simulink model "lab_1_v3"  (R2014a)
settings: Solver=ode3  StartTime=0.0  StopTime=inf  RelTol=1e-3
values from neighbouring files (symbols this model uses):
  a = 1    [aaa.m]    (also in forward.m = ai(i); forward_inverse.m = ai(i); init.m = [0 l 0 0 0 0]; inverse.m = ai(i))
  al = [90 0 -90 90 -90 0]    [init.m]    (also in inverse.m = [pi/2 0 -pi/2 pi/2 -pi/2 0])
  d = di(i)    [forward.m]    (also in forward_inverse.m; init.m = [l 0 0 2*l 0 2*l]; inverse.m; lab_1.m)
  s = zc - d(1)    [inverse.m]
  simout = [0 0 0; 0 0 0; 0 0 0]    [init.m]
libraries: mblibv1 x26, simulink x6
settings Model: Creator=kirix  LastModifiedBy=kirix
settings SimMechanicsCC: VisDuringSimulation=on

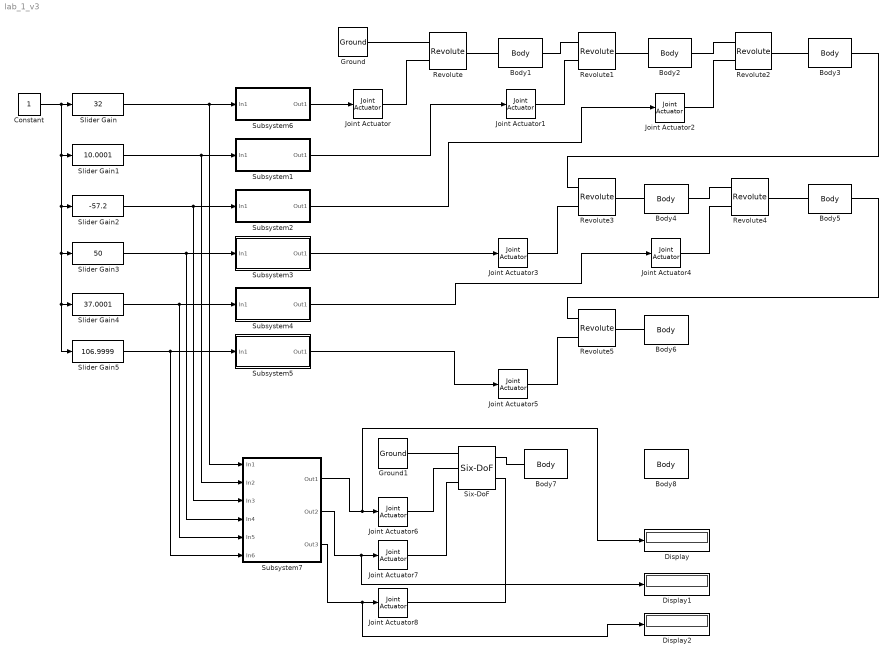
== system lab_1_v3 ==
  Body1 : mblibv1/Bodies/Body  LConnTagsString=CS1  RConnTagsString=CS2  UpdateFromCAD=off  DialogClass=MechanicalBodyBlock  Mass=1  MassUnits=kg  InertiaUnits=kg*m^2  Inertia=eye(3)  Shape=Cylinder  ShapeDims=[1 1]  ShapeUnits=m  ShapeUse=false  Density=1  DensityUnits=kg/m^3  DensityUse=false  GraphicsMode=MACHINE_DEFAULT  BodyColorSelMode=MACHINE_DEFAULT  BodyColor=[1 0 0]  AttachedToCS=CG  CG=Left$CG$[0 0 0]$CS1$CS1$m$[0 0 0]$Euler X-Y-Z$deg$CS1$false$none  WorkingFrames=Left$CS1$[0 0 0]$Adjoining$Adjoining$m$[0 0 0]$Euler X-Y-Z$deg$Adjoining$true$none#Right$CS2$[0 0 d(1)]$CS1$CS1$m$[al(1) 0 0]$Euler X-Y-Z$deg$CS1$true$none  CGPos=[0 0 0]  CGRot=[0 0 0]  CS0Pos=[]  CS0Rot=[]  CS1Pos=[0 0 0]  CS1Rot=[0 0 0]  CS2Pos=[0 0 d(1)]  CS2Rot=[al(1) 0 0]  CS3Pos=[]  CS3Rot=[]  CS4Pos=[]  CS4Rot=[]  CS5Pos=[]  CS5Rot=[]  CS6Pos=[]  CS6Rot=[]  CS7Pos=[]  CS7Rot=[]  CS8Pos=[]  CS8Rot=[]  CS9Pos=[]  CS9Rot=[]  CS10Pos=[]  CS10Rot=[]  CS11Pos=[]  CS11Rot=[]  CS12Pos=[]  CS12Rot=[]  CS13Pos=[]  CS13Rot=[]  CS14Pos=[]  CS14Rot=[]  CS15Pos=[]  CS15Rot=[]  CS16Pos=[]  CS16Rot=[]  CS17Pos=[]  CS17Rot=[]  CS18Pos=[]  CS18Rot=[]  CS19Pos=[]  CS19Rot=[]  CS20Pos=[]  CS20Rot=[]
  Body2 : mblibv1/Bodies/Body  LConnTagsString=CS1  RConnTagsString=CS2  UpdateFromCAD=off  DialogClass=MechanicalBodyBlock  Mass=1  MassUnits=kg  InertiaUnits=kg*m^2  Inertia=eye(3)  Shape=Cylinder  ShapeDims=[1 1]  ShapeUnits=m  ShapeUse=false  Density=1  DensityUnits=kg/m^3  DensityUse=false  GraphicsMode=MACHINE_DEFAULT  BodyColorSelMode=MACHINE_DEFAULT  BodyColor=[1 0 0]  AttachedToCS=CG  CG=Left$CG$[0 0 0]$CS1$CS1$m$[0 0 0]$Euler X-Y-Z$deg$CS1$false$none  WorkingFrames=Left$CS1$[0 0 0]$Adjoining$Adjoining$m$[0 0 0]$Euler X-Y-Z$deg$Adjoining$true$none#Right$CS2$[a(2) 0 0]$CS1$CS1$m$[0 0 0]$Euler X-Y-Z$deg$CS1$true$none  CGPos=[0 0 0]  CGRot=[0 0 0]  CS0Pos=[]  CS0Rot=[]  CS1Pos=[0 0 0]  CS1Rot=[0 0 0]  CS2Pos=[a(2) 0 0]  CS2Rot=[0 0 0]  CS3Pos=[]  CS3Rot=[]  CS4Pos=[]  CS4Rot=[]  CS5Pos=[]  CS5Rot=[]  CS6Pos=[]  CS6Rot=[]  CS7Pos=[]  CS7Rot=[]  CS8Pos=[]  CS8Rot=[]  CS9Pos=[]  CS9Rot=[]  CS10Pos=[]  CS10Rot=[]  CS11Pos=[]  CS11Rot=[]  CS12Pos=[]  CS12Rot=[]  CS13Pos=[]  CS13Rot=[]  CS14Pos=[]  CS14Rot=[]  CS15Pos=[]  CS15Rot=[]  CS16Pos=[]  CS16Rot=[]  CS17Pos=[]  CS17Rot=[]  CS18Pos=[]  CS18Rot=[]  CS19Pos=[]  CS19Rot=[]  CS20Pos=[]  CS20Rot=[]
  Body3 : mblibv1/Bodies/Body  LConnTagsString=CS1  RConnTagsString=CS2  UpdateFromCAD=off  DialogClass=MechanicalBodyBlock  Mass=1  MassUnits=kg  InertiaUnits=kg*m^2  Inertia=eye(3)  Shape=Cylinder  ShapeDims=[1 1]  ShapeUnits=m  ShapeUse=false  Density=1  DensityUnits=kg/m^3  DensityUse=false  GraphicsMode=MACHINE_DEFAULT  BodyColorSelMode=MACHINE_DEFAULT  BodyColor=[1 0 0]  AttachedToCS=CG  CG=Left$CG$[0 0 0]$CS1$CS1$m$[0 0 0]$Euler X-Y-Z$deg$CS1$false$none  WorkingFrames=Left$CS1$[0 0 0]$Adjoining$Adjoining$m$[0 0 0]$Euler X-Y-Z$deg$Adjoining$true$none#Right$CS2$[0 0 d(3)]$CS1$CS1$m$[al(3) 0 0]$Euler X-Y-Z$deg$CS1$true$none  CGPos=[0 0 0]  CGRot=[0 0 0]  CS0Pos=[]  CS0Rot=[]  CS1Pos=[0 0 0]  CS1Rot=[0 0 0]  CS2Pos=[0 0 d(3)]  CS2Rot=[al(3) 0 0]  CS3Pos=[]  CS3Rot=[]  CS4Pos=[]  CS4Rot=[]  CS5Pos=[]  CS5Rot=[]  CS6Pos=[]  CS6Rot=[]  CS7Pos=[]  CS7Rot=[]  CS8Pos=[]  CS8Rot=[]  CS9Pos=[]  CS9Rot=[]  CS10Pos=[]  CS10Rot=[]  CS11Pos=[]  CS11Rot=[]  CS12Pos=[]  CS12Rot=[]  CS13Pos=[]  CS13Rot=[]  CS14Pos=[]  CS14Rot=[]  CS15Pos=[]  CS15Rot=[]  CS16Pos=[]  CS16Rot=[]  CS17Pos=[]  CS17Rot=[]  CS18Pos=[]  CS18Rot=[]  CS19Pos=[]  CS19Rot=[]  CS20Pos=[]  CS20Rot=[]
  Body4 : mblibv1/Bodies/Body  LConnTagsString=CS1  RConnTagsString=CS2  UpdateFromCAD=off  DialogClass=MechanicalBodyBlock  Mass=1  MassUnits=kg  InertiaUnits=kg*m^2  Inertia=eye(3)  Shape=Cylinder  ShapeDims=[1 1]  ShapeUnits=m  ShapeUse=false  Density=1  DensityUnits=kg/m^3  DensityUse=false  GraphicsMode=MACHINE_DEFAULT  BodyColorSelMode=MACHINE_DEFAULT  BodyColor=[1 0 0]  AttachedToCS=CG  CG=Left$CG$[0 0 0]$CS1$CS1$m$[0 0 0]$Euler X-Y-Z$deg$CS1$false$none  WorkingFrames=Left$CS1$[0 0 0]$Adjoining$Adjoining$m$[0 0 0]$Euler X-Y-Z$deg$Adjoining$true$none#Right$CS2$[0 0 d(4)]$CS1$CS1$m$[al(4) 0 0]$Euler X-Y-Z$deg$CS1$true$none  CGPos=[0 0 0]  CGRot=[0 0 0]  CS0Pos=[]  CS0Rot=[]  CS1Pos=[0 0 0]  CS1Rot=[0 0 0]  CS2Pos=[0 0 d(4)]  CS2Rot=[al(4) 0 0]  CS3Pos=[]  CS3Rot=[]  CS4Pos=[]  CS4Rot=[]  CS5Pos=[]  CS5Rot=[]  CS6Pos=[]  CS6Rot=[]  CS7Pos=[]  CS7Rot=[]  CS8Pos=[]  CS8Rot=[]  CS9Pos=[]  CS9Rot=[]  CS10Pos=[]  CS10Rot=[]  CS11Pos=[]  CS11Rot=[]  CS12Pos=[]  CS12Rot=[]  CS13Pos=[]  CS13Rot=[]  CS14Pos=[]  CS14Rot=[]  CS15Pos=[]  CS15Rot=[]  CS16Pos=[]  CS16Rot=[]  CS17Pos=[]  CS17Rot=[]  CS18Pos=[]  CS18Rot=[]  CS19Pos=[]  CS19Rot=[]  CS20Pos=[]  CS20Rot=[]
  Body5 : mblibv1/Bodies/Body  LConnTagsString=CS1  RConnTagsString=CS2  UpdateFromCAD=off  DialogClass=MechanicalBodyBlock  Mass=1  MassUnits=kg  InertiaUnits=kg*m^2  Inertia=eye(3)  Shape=Cylinder  ShapeDims=[1 1]  ShapeUnits=m  ShapeUse=false  Density=1  DensityUnits=kg/m^3  DensityUse=false  GraphicsMode=MACHINE_DEFAULT  BodyColorSelMode=MACHINE_DEFAULT  BodyColor=[1 0 0]  AttachedToCS=CG  CG=Left$CG$[0 0 0]$CS1$CS1$m$[0 0 0]$Euler X-Y-Z$deg$CS1$false$none  WorkingFrames=Left$CS1$[0 0 0]$Adjoining$Adjoining$m$[0 0 0]$Euler X-Y-Z$deg$Adjoining$true$none#Right$CS2$[0 0 d(5)]$CS1$CS1$m$[al(5) 0 0]$Euler X-Y-Z$deg$CS1$true$none  CGPos=[0 0 0]  CGRot=[0 0 0]  CS0Pos=[]  CS0Rot=[]  CS1Pos=[0 0 0]  CS1Rot=[0 0 0]  CS2Pos=[0 0 d(5)]  CS2Rot=[al(5) 0 0]  CS3Pos=[]  CS3Rot=[]  CS4Pos=[]  CS4Rot=[]  CS5Pos=[]  CS5Rot=[]  CS6Pos=[]  CS6Rot=[]  CS7Pos=[]  CS7Rot=[]  CS8Pos=[]  CS8Rot=[]  CS9Pos=[]  CS9Rot=[]  CS10Pos=[]  CS10Rot=[]  CS11Pos=[]  CS11Rot=[]  CS12Pos=[]  CS12Rot=[]  CS13Pos=[]  CS13Rot=[]  CS14Pos=[]  CS14Rot=[]  CS15Pos=[]  CS15Rot=[]  CS16Pos=[]  CS16Rot=[]  CS17Pos=[]  CS17Rot=[]  CS18Pos=[]  CS18Rot=[]  CS19Pos=[]  CS19Rot=[]  CS20Pos=[]  CS20Rot=[]
  Body6 : mblibv1/Bodies/Body  LConnTagsString=CS1  RConnTagsString=CS2  UpdateFromCAD=off  DialogClass=MechanicalBodyBlock  Mass=1  MassUnits=kg  InertiaUnits=kg*m^2  Inertia=eye(3)  Shape=Cylinder  ShapeDims=[1 1]  ShapeUnits=m  ShapeUse=false  Density=1  DensityUnits=kg/m^3  DensityUse=false  GraphicsMode=MACHINE_DEFAULT  BodyColorSelMode=MACHINE_DEFAULT  BodyColor=[1 0 0]  AttachedToCS=CG  CG=Left$CG$[0 0 0]$CS1$CS1$m$[0 0 0]$Euler X-Y-Z$deg$CS1$false$none  WorkingFrames=Left$CS1$[0 0 0]$Adjoining$Adjoining$m$[0 0 0]$Euler X-Y-Z$deg$Adjoining$true$none#Right$CS2$[0 0 d(6)]$CS1$CS1$m$[0 0 0]$Euler X-Y-Z$deg$CS1$true$none  CGPos=[0 0 0]  CGRot=[0 0 0]  CS0Pos=[]  CS0Rot=[]  CS1Pos=[0 0 0]  CS1Rot=[0 0 0]  CS2Pos=[0 0 d(6)]  CS2Rot=[0 0 0]  CS3Pos=[]  CS3Rot=[]  CS4Pos=[]  CS4Rot=[]  CS5Pos=[]  CS5Rot=[]  CS6Pos=[]  CS6Rot=[]  CS7Pos=[]  CS7Rot=[]  CS8Pos=[]  CS8Rot=[]  CS9Pos=[]  CS9Rot=[]  CS10Pos=[]  CS10Rot=[]  CS11Pos=[]  CS11Rot=[]  CS12Pos=[]  CS12Rot=[]  CS13Pos=[]  CS13Rot=[]  CS14Pos=[]  CS14Rot=[]  CS15Pos=[]  CS15Rot=[]  CS16Pos=[]  CS16Rot=[]  CS17Pos=[]  CS17Rot=[]  CS18Pos=[]  CS18Rot=[]  CS19Pos=[]  CS19Rot=[]  CS20Pos=[]  CS20Rot=[]
  Body7 : mblibv1/Bodies/Body  LConnTagsString=CS1  RConnTagsString=CS2  UpdateFromCAD=off  DialogClass=MechanicalBodyBlock  Mass=1  MassUnits=kg  InertiaUnits=kg*m^2  Inertia=eye(3)  Shape=Cylinder  ShapeDims=[1 1]  ShapeUnits=m  ShapeUse=false  Density=1  DensityUnits=kg/m^3  DensityUse=false  GraphicsMode=MACHINE_DEFAULT  BodyColorSelMode=MACHINE_DEFAULT  BodyColor=[1 0 0]  AttachedToCS=CG  CG=Left$CG$[0 0 0]$CS1$CS1$m$[0 0 0]$Euler X-Y-Z$deg$CS1$false$none  WorkingFrames=Left$CS1$[0 0 0]$Adjoining$Adjoining$m$[0 0 0]$Euler X-Y-Z$deg$Adjoining$true$none#Right$CS2$[0 0 2]$CS1$CS1$m$[0 0 0]$Euler X-Y-Z$deg$CS1$true$none  CGPos=[0 0 0]  CGRot=[0 0 0]  CS0Pos=[]  CS0Rot=[]  CS1Pos=[0 0 0]  CS1Rot=[0 0 0]  CS2Pos=[0 0 2]  CS2Rot=[0 0 0]  CS3Pos=[]  CS3Rot=[]  CS4Pos=[]  CS4Rot=[]  CS5Pos=[]  CS5Rot=[]  CS6Pos=[]  CS6Rot=[]  CS7Pos=[]  CS7Rot=[]  CS8Pos=[]  CS8Rot=[]  CS9Pos=[]  CS9Rot=[]  CS10Pos=[]  CS10Rot=[]  CS11Pos=[]  CS11Rot=[]  CS12Pos=[]  CS12Rot=[]  CS13Pos=[]  CS13Rot=[]  CS14Pos=[]  CS14Rot=[]  CS15Pos=[]  CS15Rot=[]  CS16Pos=[]  CS16Rot=[]  CS17Pos=[]  CS17Rot=[]  CS18Pos=[]  CS18Rot=[]  CS19Pos=[]  CS19Rot=[]  CS20Pos=[]  CS20Rot=[]
  Body8 : mblibv1/Bodies/Body  LConnTagsString=CS1  RConnTagsString=CS2  UpdateFromCAD=off  DialogClass=MechanicalBodyBlock  Mass=1  MassUnits=kg  InertiaUnits=kg*m^2  Inertia=eye(3)  Shape=Cylinder  ShapeDims=[1 1]  ShapeUnits=m  ShapeUse=false  Density=1  DensityUnits=kg/m^3  DensityUse=false  GraphicsMode=MACHINE_DEFAULT  BodyColorSelMode=MACHINE_DEFAULT  BodyColor=[1 0 0]  AttachedToCS=CG  CG=Left$CG$[0 0 0]$CS1$CS1$m$[0 0 0]$Euler X-Y-Z$deg$CS1$false$none  WorkingFrames=Left$CS1$[0 0 0]$Adjoining$Adjoining$m$[0 0 0]$Euler X-Y-Z$deg$Adjoining$true$none#Right$CS2$[simout(1,1) simout(1,2) simout(1,3)]$CS1$CS1$m$[0 0 0]$Euler X-Y-Z$deg$CS1$true$none  CGPos=[0 0 0]  CGRot=[0 0 0]  CS0Pos=[]  CS0Rot=[]  CS1Pos=[0 0 0]  CS1Rot=[0 0 0]  CS2Pos=[simout(1,1) simout(1,2) simout(1,3)]  CS2Rot=[0 0 0]  CS3Pos=[]  CS3Rot=[]  CS4Pos=[]  CS4Rot=[]  CS5Pos=[]  CS5Rot=[]  CS6Pos=[]  CS6Rot=[]  CS7Pos=[]  CS7Rot=[]  CS8Pos=[]  CS8Rot=[]  CS9Pos=[]  CS9Rot=[]  CS10Pos=[]  CS10Rot=[]  CS11Pos=[]  CS11Rot=[]  CS12Pos=[]  CS12Rot=[]  CS13Pos=[]  CS13Rot=[]  CS14Pos=[]  CS14Rot=[]  CS15Pos=[]  CS15Rot=[]  CS16Pos=[]  CS16Rot=[]  CS17Pos=[]  CS17Rot=[]  CS18Pos=[]  CS18Rot=[]  CS19Pos=[]  CS19Rot=[]  CS20Pos=[]  CS20Rot=[]
  Constant : Constant
  Display : Display
  Display1 : Display
  Display2 : Display
  Ground : mblibv1/Bodies/Ground  UpdateFromCAD=off  LeftPortType=env  RightPortType=workingframe  PhysicalDomain=Mechanical  DialogClass=GroundBlock  CoordPosition=[0 0 0]  CoordPositionUnits=m  StateVectorMgrId=11  MachineId=[6 1]  ShowEnvPort=off  ParameterChecksum=[3934137374, 916383386, 1487276708, 2248275688]  TopologyChecksum=[3248512813, 3168158489, 2501519655, 3439787685]
  Ground1 : mblibv1/Bodies/Ground  UpdateFromCAD=off  LeftPortType=env  RightPortType=workingframe  PhysicalDomain=Mechanical  DialogClass=GroundBlock  CoordPosition=[0 0 0]  CoordPositionUnits=m  StateVectorMgrId=12  MachineId=[6 2]  ShowEnvPort=off  ParameterChecksum=[2997898288, 4175519526, 3238191346, 431706980]  TopologyChecksum=[1840042938, 3660248777, 934597290, 2913613180]
  Joint Actuator{,1..5} (6 alike) : mblibv1/Sensors &  Actuators/Joint Actuator  UpdateFromCAD=off  PhysicalDomain=Mechanical  PortType=blob  ActuationStyle=Motion  AngleUnits=deg  ArcVelocityUnits=deg/s  ArcAccelerationUnits=deg/s^2  CoordPositionUnits=m  VelocityUnits=m/s  AccelerationUnits=m/s^2  ForceUnits=N  TorqueUnits=N*m  ActiveIO=on  Width=3  DialogClass=MechanicalActuatorBlock  Primitive=R1  ReferenceFrame=Absolute (World)
  Joint Actuator6 : mblibv1/Sensors &  Actuators/Joint Actuator  UpdateFromCAD=off  PhysicalDomain=Mechanical  PortType=blob  ActuationStyle=Motion  AngleUnits=deg  ArcVelocityUnits=deg/s  ArcAccelerationUnits=deg/s^2  CoordPositionUnits=m  VelocityUnits=m/s  AccelerationUnits=m/s^2  ForceUnits=N  TorqueUnits=N*m  ActiveIO=on  Width=3  DialogClass=MechanicalActuatorBlock  Primitive=P1  ReferenceFrame=Absolute (World)
  Joint Actuator7 : mblibv1/Sensors &  Actuators/Joint Actuator  UpdateFromCAD=off  PhysicalDomain=Mechanical  PortType=blob  ActuationStyle=Motion  AngleUnits=deg  ArcVelocityUnits=deg/s  ArcAccelerationUnits=deg/s^2  CoordPositionUnits=m  VelocityUnits=m/s  AccelerationUnits=m/s^2  ForceUnits=N  TorqueUnits=N*m  ActiveIO=on  Width=3  DialogClass=MechanicalActuatorBlock  Primitive=P2  ReferenceFrame=Absolute (World)
  Joint Actuator8 : mblibv1/Sensors &  Actuators/Joint Actuator  UpdateFromCAD=off  PhysicalDomain=Mechanical  PortType=blob  ActuationStyle=Motion  AngleUnits=deg  ArcVelocityUnits=deg/s  ArcAccelerationUnits=deg/s^2  CoordPositionUnits=m  VelocityUnits=m/s  AccelerationUnits=m/s^2  ForceUnits=N  TorqueUnits=N*m  ActiveIO=on  Width=3  DialogClass=MechanicalActuatorBlock  Primitive=P3  ReferenceFrame=Absolute (World)
  Revolute : mblibv1/Joints/Revolute  LConnTagsString=__newl0|SA1  RConnTagsString=__newr0  UpdateFromCAD=off  NumSAPorts=1  CutJoint=on  MarkAsCut=off  Primitives=prismatic  PrimitiveProps=R1$Base$[0 0 1]$revolute  DialogClass=JointBlock  R1Axis=[0 0 1]
  Revolute{1..5} (5 alike) : mblibv1/Joints/Revolute  LConnTagsString=__newl0|SA1  RConnTagsString=__newr0  UpdateFromCAD=off  NumSAPorts=1  CutJoint=off  MarkAsCut=off  Primitives=prismatic  PrimitiveProps=R1$Base$[0 0 1]$revolute  DialogClass=JointBlock  R1Axis=[0 0 1]
  Six-DoF : mblibv1/Joints/Six-DoF  LConnTagsString=__newl0|SA1|SA2  RConnTagsString=__newr0|SA1  UpdateFromCAD=off  NumSAPorts=3  CutJoint=off  MarkAsCut=off  Primitives=prismatic_prismatic  PrimitiveProps=P1$Follower$[1 0 0]$prismatic#P2$Follower$[0 1 0]$prismatic#P3$Follower$[0 0 1]$prismatic#S$World$[0 0 0]$spherical  DialogClass=JointBlock  P1Axis=[1 0 0]  P2Axis=[0 1 0]  P3Axis=[0 0 1]  SAxis=[0 0 0]
  Slider Gain : simulink/Math Operations/Slider Gain  Tag=sg1  low=-180  gain=32  high=180
  Slider Gain1 : simulink/Math Operations/Slider Gain  low=-180  gain=10.0001  high=180
  Slider Gain2 : simulink/Math Operations/Slider Gain  low=-180  gain=-57.2  high=180
  Slider Gain3 : simulink/Math Operations/Slider Gain  low=-180  gain=50  high=180
  Slider Gain4 : simulink/Math Operations/Slider Gain  low=-180  gain=37.0001  high=180
  Slider Gain5 : simulink/Math Operations/Slider Gain  low=-180  gain=106.9999  high=180
  Subsystem1 : Subsystem
  Subsystem2 : Subsystem
  Subsystem3 : Subsystem
  Subsystem4 : Subsystem
  Subsystem5 : Subsystem
  Subsystem6 : Subsystem
  Subsystem7 : Subsystem
  wires:
  Slider Gain/1 -> Subsystem7/1(In1), Subsystem6/1(In1)
  Slider Gain1/1 -> Subsystem7/2(In2), Subsystem1/1(In1)
  Subsystem1/1(Out1) -> Joint Actuator1/1
  Slider Gain2/1 -> Subsystem7/3(In3), Subsystem2/1(In1)
  Subsystem2/1(Out1) -> Joint Actuator2/1
  Slider Gain3/1 -> Subsystem7/4(In4), Subsystem3/1(In1)
  Subsystem3/1(Out1) -> Joint Actuator3/1
  Slider Gain4/1 -> Subsystem7/5(In5), Subsystem4/1(In1)
  Subsystem4/1(Out1) -> Joint Actuator4/1
  Slider Gain5/1 -> Subsystem7/6(In6), Subsystem5/1(In1)
  Subsystem5/1(Out1) -> Joint Actuator5/1
  Constant/1 -> Slider Gain5/1, Slider Gain4/1, Slider Gain3/1, Slider Gain2/1, Slider Gain1/1, Slider Gain/1
  Subsystem6/1(Out1) -> Joint Actuator/1
  Subsystem7/1(Out1) -> Display/1, Joint Actuator6/1
  Subsystem7/2(Out2) -> Display1/1, Joint Actuator7/1
  Subsystem7/3(Out3) -> Display2/1, Joint Actuator8/1
  connections:
  Ground/RConn1 -- Revolute/LConn1
  Body1/LConn1 -- Revolute/RConn1
  Joint Actuator1/RConn1 -- Revolute1/LConn2
  Joint Actuator2/RConn1 -- Revolute2/LConn2
  Revolute2/LConn1 -- Body2/RConn1
  Revolute1/RConn1 -- Body2/LConn1
  Revolute2/RConn1 -- Body3/LConn1
  Joint Actuator3/RConn1 -- Revolute3/LConn2
  Revolute3/LConn1 -- Body3/RConn1
  Revolute3/RConn1 -- Body4/LConn1
  Joint Actuator4/RConn1 -- Revolute4/LConn2
  Revolute4/LConn1 -- Body4/RConn1
  Revolute4/RConn1 -- Body5/LConn1
  Joint Actuator5/RConn1 -- Revolute5/LConn2
  Revolute5/LConn1 -- Body5/RConn1
  Revolute5/RConn1 -- Body6/LConn1
  Joint Actuator/RConn1 -- Revolute/LConn2
  Body1/RConn1 -- Revolute1/LConn1
  Six-DoF/RConn1 -- Body7/LConn1
  Ground1/RConn1 -- Six-DoF/LConn1
  Joint Actuator6/RConn1 -- Six-DoF/LConn2
  Joint Actuator7/RConn1 -- Six-DoF/LConn3
  Joint Actuator8/RConn1 -- Six-DoF/RConn2

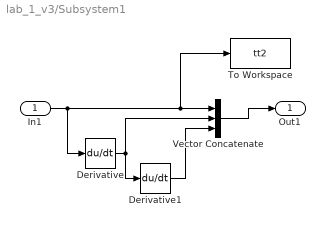
== system lab_1_v3/Subsystem1 ==
  In1 : Inport
  Derivative : Derivative
  Derivative1 : Derivative
  To Workspace : ToWorkspace  VariableName=tt2  SampleTime=-1
      settings: Save2DSignal=2-D array (concatenate along first dimension)
  Vector Concatenate : Concatenate  NumInputs=3
  Out1 : Outport  PortDimensions=3
  wires:
  In1/1 -> To Workspace/1, Vector Concatenate/1, Derivative/1
  Derivative/1 -> Vector Concatenate/2, Derivative1/1
  Derivative1/1 -> Vector Concatenate/3
  Vector Concatenate/1 -> Out1/1

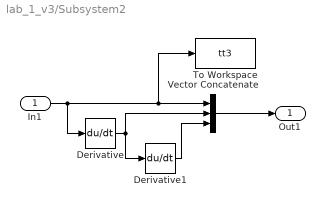
== system lab_1_v3/Subsystem2 ==
  In1 : Inport
  Derivative : Derivative
  Derivative1 : Derivative
  To Workspace : ToWorkspace  VariableName=tt3  SampleTime=-1
      settings: Save2DSignal=2-D array (concatenate along first dimension)
  Vector Concatenate : Concatenate  NumInputs=3
  Out1 : Outport  PortDimensions=3
  wires:
  In1/1 -> To Workspace/1, Vector Concatenate/1, Derivative/1
  Derivative1/1 -> Vector Concatenate/3
  Derivative/1 -> Vector Concatenate/2, Derivative1/1
  Vector Concatenate/1 -> Out1/1

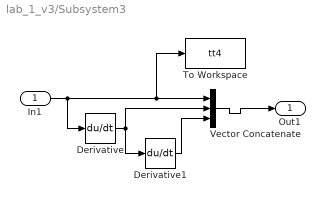
== system lab_1_v3/Subsystem3 ==
  In1 : Inport
  Derivative : Derivative
  Derivative1 : Derivative
  To Workspace : ToWorkspace  VariableName=tt4  SampleTime=-1
      settings: Save2DSignal=2-D array (concatenate along first dimension)
  Vector Concatenate : Concatenate  NumInputs=3
  Out1 : Outport  PortDimensions=3
  wires:
  In1/1 -> To Workspace/1, Vector Concatenate/1, Derivative/1
  Derivative/1 -> Vector Concatenate/2, Derivative1/1
  Vector Concatenate/1 -> Out1/1
  Derivative1/1 -> Vector Concatenate/3

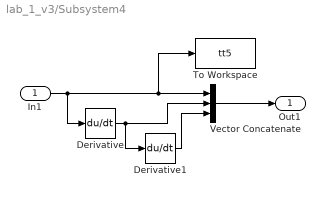
== system lab_1_v3/Subsystem4 ==
  In1 : Inport
  Derivative : Derivative
  Derivative1 : Derivative
  To Workspace : ToWorkspace  VariableName=tt5  SampleTime=-1
      settings: Save2DSignal=2-D array (concatenate along first dimension)
  Vector Concatenate : Concatenate  NumInputs=3
  Out1 : Outport  PortDimensions=3
  wires:
  In1/1 -> To Workspace/1, Vector Concatenate/1, Derivative/1
  Derivative1/1 -> Vector Concatenate/3
  Derivative/1 -> Vector Concatenate/2, Derivative1/1
  Vector Concatenate/1 -> Out1/1

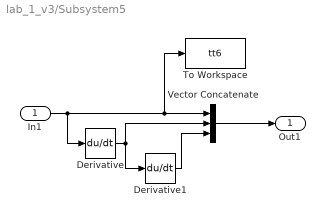
== system lab_1_v3/Subsystem5 ==
  In1 : Inport
  Derivative : Derivative
  Derivative1 : Derivative
  To Workspace : ToWorkspace  VariableName=tt6  SampleTime=-1
      settings: Save2DSignal=2-D array (concatenate along first dimension)
  Vector Concatenate : Concatenate  NumInputs=3
  Out1 : Outport  PortDimensions=3
  wires:
  In1/1 -> To Workspace/1, Vector Concatenate/1, Derivative/1
  Derivative1/1 -> Vector Concatenate/3
  Derivative/1 -> Derivative1/1, Vector Concatenate/2
  Vector Concatenate/1 -> Out1/1

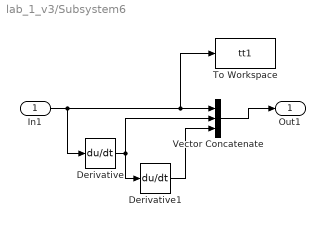
== system lab_1_v3/Subsystem6 ==
  In1 : Inport
  Derivative : Derivative
  Derivative1 : Derivative
  To Workspace : ToWorkspace  VariableName=tt1  SampleTime=-1
      settings: Save2DSignal=2-D array (concatenate along first dimension)
  Vector Concatenate : Concatenate  NumInputs=3  ConcatenateDimension=3
  Out1 : Outport  PortDimensions=3
  wires:
  In1/1 -> To Workspace/1, Vector Concatenate/1, Derivative/1
  Derivative/1 -> Vector Concatenate/2, Derivative1/1
  Derivative1/1 -> Vector Concatenate/3
  Vector Concatenate/1 -> Out1/1

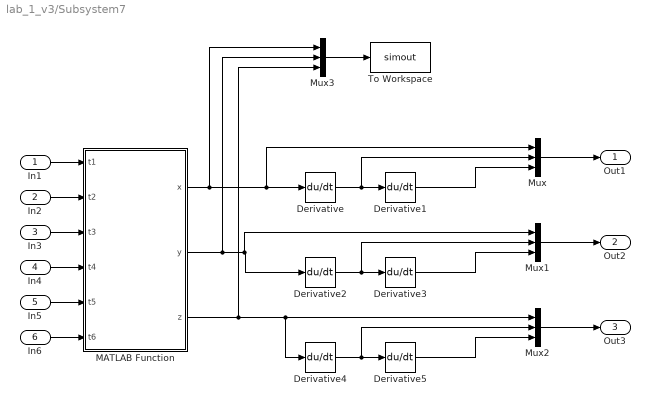
== system lab_1_v3/Subsystem7 ==
  In1 : Inport
  In2 : Inport  Port=2
  In3 : Inport  Port=3
  In4 : Inport  Port=4
  In5 : Inport  Port=5
  In6 : Inport  Port=6
  Derivative{,1..5} (6 alike) : Derivative
  MATLAB Function : MATLAB Function  TreatAsAtomicUnit=on
  Mux{,1..3} (4 alike) : Mux  Inputs=3
  To Workspace : ToWorkspace  VariableName=simout  SampleTime=-1
  Out1 : Outport  PortDimensions=3
  Out2 : Outport  Port=2  PortDimensions=3
  Out3 : Outport  Port=3  PortDimensions=3
  wires:
  In1/1 -> MATLAB Function/1(t1)
  In2/1 -> MATLAB Function/2(t2)
  In3/1 -> MATLAB Function/3(t3)
  In4/1 -> MATLAB Function/4(t4)
  In5/1 -> MATLAB Function/5(t5)
  In6/1 -> MATLAB Function/6(t6)
  Mux/1 -> Out1/1
  Derivative/1 -> Derivative1/1, Mux/2
  Derivative1/1 -> Mux/3
  Mux1/1 -> Out2/1
  Derivative2/1 -> Derivative3/1, Mux1/2
  Derivative3/1 -> Mux1/3
  Mux2/1 -> Out3/1
  Derivative4/1 -> Derivative5/1, Mux2/2
  Derivative5/1 -> Mux2/3
  MATLAB Function/3(z) -> Mux3/3, Mux2/1, Derivative4/1
  MATLAB Function/1(x) -> Mux3/1, Mux/1, Derivative/1
  MATLAB Function/2(y) -> Mux3/2, Mux1/1, Derivative2/1
  Mux3/1 -> To Workspace/1

== matlab function lab_1_v3/Subsystem7/MATLAB Function ==
  data: x output; t1 input; y output; t2 input; t3 input; t4 input; t5 input; t6 input; z output
function [x,y,z] = fcn(t1, t2, t3, t4, t5, t6)
    %#codegen
    l = 10;
    angle = pi / 2;

    tetta = [t1 t2 t3 t4 t5 t6];
    di =    [l 0 0 2*l 0 2*l];
    ai =    [0 l 0 0 0 0];
    alpha = [angle 0 -angle angle -angle 0];

    H = [
        1 0 0 0;
        0 1 0 0;
        0 0 1 0;
        0 0 0 1;
    ];

    for i = 1:6
        c_t = cos(tetta(i)*pi/180);
        s_t = sin(tetta(i)*pi/180);
        d = di(i);
        a = ai(i);
        c_a = cos(alpha(i));
        s_a = sin(alpha(i));

        Rtz = [
            c_t -s_t 0 0;
            s_t c_t 0 0;
            0 0 1 0;
            0 0 0 1
        ];
        Tz = [
            1 0 0 0;
            0 1 0 0;
            0 0 1 d;
            0 0 0 1
        ];
        Tx = [
            1 0 0 a;
            0 1 0 0;
            0 0 1 0;
            0 0 0 1
        ];
        Rtx = [
            1 0 0 0;
            0 c_a -s_a 0;
            0 s_a c_a 0;
            0 0 0 1
        ];

        A = Rtz * Tz * Tx * Rtx;
        H = H * A;
    end

    x = H(1, 4);
    y = H(2, 4);
    z = H(3, 4);

end
